simulink model "model_obsr"  (R2022b)
settings: Solver=ode4  StartTime=0.0  StopTime=100  FixedStep=time_step  RelTol=1e-3
values from neighbouring files (symbols this model uses):
  G1_vec = []    [initialization.m]
  G2_vec = []    [initialization.m]
  n = length(A)    [initialization.m]    (also in qualityfactor.m)
  time_samples_count = length(time_stamps)    [initialization.m]
  time_stamps = 0 : time_step :T    [initialization.m]
  time_step = 0.01    [initialization.m]
  x0 = [0 0]    [initialization.m]
undefined symbols (not defined in the file or in its folder): A, B, C
libraries: simulink x4
settings Model: Creator=Ja  LastModifiedBy=Ja

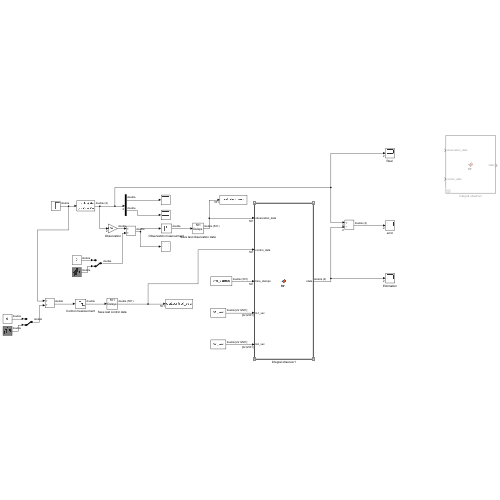
[thumbnail: Simulink's stored preview of the top-level diagram]
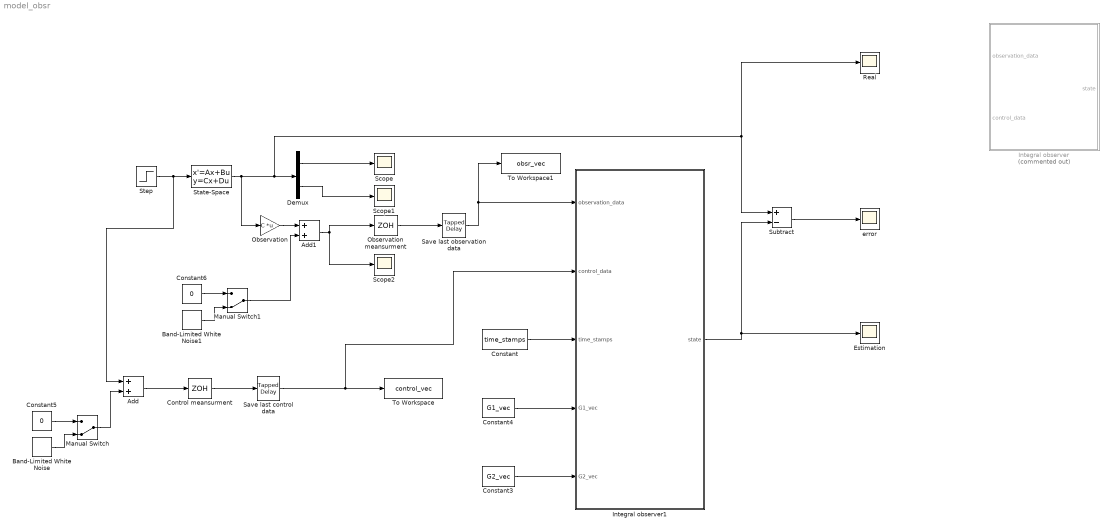
== system model_obsr ==
  Add : Sum
  Add1 : Sum
  Band-Limited White Noise : simulink/Sources/Band-Limited White Noise  Cov=[0.001]  Ts=time_step  seed=[23341]
  Band-Limited White Noise1 : simulink/Sources/Band-Limited White Noise  Cov=[0.001]  Ts=time_step  seed=[23341]
  Constant : Constant  Value=time_stamps
  Constant3 : Constant  Value=G2_vec
  Constant4 : Constant  Value=G1_vec
  Constant5 : Constant  Value=0
  Constant6 : Constant  Value=0
  Control meansurment : ZeroOrderHold  SampleTime=time_step
  Demux : Demux  Outputs=2
  Estimation : Scope
  Integral observer : MATLAB Function  Commented=on  TreatAsAtomicUnit=on
  Integral observer1 : MATLAB Function  TreatAsAtomicUnit=on
  Manual Switch : ManualSwitch  CurrentSetting=0
  Manual Switch1 : ManualSwitch  CurrentSetting=0
  Observation : Gain  Gain=C  Multiplication=Matrix(K*u)
  Observation meansurment : ZeroOrderHold  SampleTime=time_step
  "Real " : Scope
  Save last control data : simulink/Discrete/Tapped Delay  vinit=0.0  samptime=-1  NumDelays=time_samples_count  DelayOrder=Oldest  includeCurrent=off
  Save last observation data : simulink/Discrete/Tapped Delay  vinit=0.0  samptime=-1  NumDelays=time_samples_count  DelayOrder=Oldest  includeCurrent=off
  Scope : Scope
  Scope1 : Scope
  Scope2 : Scope
  State-Space : StateSpace  A=A  B=B  C=diag(ones([n 1]))  D=zeros([2 1])  InitialCondition=x0
  Step : Step  SampleTime=0
  Subtract : Sum  Inputs=+-
  To Workspace : ToWorkspace  VariableName=control_vec  SampleTime=-1
  To Workspace1 : ToWorkspace  VariableName=obsr_vec  SampleTime=-1
  error : Scope
  wires:
  Observation meansurment/1 -> Save last observation data/1
  Step/1 -> Add/1, State-Space/1
  Constant3/1 -> Integral observer1/5(G2_vec)
  Save last control data/1 -> Integral observer1/2(control_data), To Workspace/1
  Control meansurment/1 -> Save last control data/1
  State-Space/1 -> "Real "/1, Subtract/1, Demux/1, Observation/1
  Demux/1 -> Scope/1
  Demux/2 -> Scope1/1
  Add1/1 -> Scope2/1, Observation meansurment/1
  Integral observer1/1(state) -> Subtract/2, Estimation/1
  Save last observation data/1 -> To Workspace1/1, Integral observer1/1(observation_data)
  Constant/1 -> Integral observer1/3(time_stamps)
  Constant4/1 -> Integral observer1/4(G1_vec)
  Subtract/1 -> error/1
  Add/1 -> Control meansurment/1
  Band-Limited White Noise/1 -> Manual Switch/2
  Constant5/1 -> Manual Switch/1
  Manual Switch/1 -> Add/2
  Band-Limited White Noise1/1 -> Manual Switch1/2
  Constant6/1 -> Manual Switch1/1
  Manual Switch1/1 -> Add1/2
  Observation/1 -> Add1/1

== matlab function model_obsr/Integral observer1 ==
  data: observation_data input; state output size=n; control_data input; time_stamps input; G1_vec input; G2_vec input
function state = fcn(observation_data, control_data, time_stamps,G1_vec, G2_vec)
%% calculate vectors
G1xY = [];
G2xU = [];
itr = 1;
for itr = 1:length(time_stamps)
    G1xY = [G1xY G1_vec(:,:, itr) * observation_data(itr)];
    G2xU = [G2xU G2_vec(:,:, itr) * control_data(itr)];
    itr = itr + 1;
end

%% make itegration of both vector
state_obs = trapz(time_stamps, G1xY, 2);
control_obs = trapz(time_stamps, G2xU, 2);

state = state_obs + control_obs;

== matlab function model_obsr/Integral observer ==
  data: observation_data input; state output; control_data input
function state = fcn(observation_data, control_data)
% load global variables
global T time_step time_stamps time_samples_count
global G1_vec G2_vec

%% calculate vectors
G1xY = [];
G2xY = [];
itr = 1;
for i = time_stamps
    G1xY(itr) = G1_vec{itr} * observation_data(itr);
    G2xY(itr) = G2_vec{itr} * control_data(itr);
    itr = itr + 1;
end


%% make itegration of both vector
state_obs = trapz(time_stamps, G1xY);
control_obs = trapz(time_stamps, G2xY);

state = state_obs + control_obs;
